simulink model "model_FS_PSH_IEEE39"  (R2020b)
settings: Solver=ode3  StartTime=0.0  StopTime=300  FixedStep=Ts  RelTol=1e-3
PostLoadFcn:
  | IEEE39BusLineLength;
  | vNomHV = 345E3;fNom=60;load('Dynamicload.mat');
InitFcn:
  | IEEE39BusLineLength;
  | vNomHV = 345E3;fNom=60;load('Dynamicload.mat');
values from neighbouring files (symbols this model uses):
  Rp = 0.05    [IEEE39BusLineLength.m]
  t_sw_off = 220    [MAIN_FS_PSH_IEEE39.m]    (also in MAIN_T_PSH_IEEE39.m; MAIN_VS_PSH.m = 45)
  t_sw_on = 130    [MAIN_FS_PSH_IEEE39.m]    (also in MAIN_T_PSH_IEEE39.m; MAIN_VS_PSH.m = 35)
  TL_10_11_len = 14    [IEEE39BusLineLength.m]
  TL_10_13_len = 14    [IEEE39BusLineLength.m]
  TL_13_14_len = 32    [IEEE39BusLineLength.m]
  TL_14_15_len = 70    [IEEE39BusLineLength.m]
  TL_15_16_len = 31.5    [IEEE39BusLineLength.m]
  TL_16_17_len = 26    [IEEE39BusLineLength.m]
  TL_16_19_len = 61    [IEEE39BusLineLength.m]
  TL_16_21_len = 46    [IEEE39BusLineLength.m]
  TL_16_24_len = 15    [IEEE39BusLineLength.m]
  TL_17_18_len = 26    [IEEE39BusLineLength.m]
  TL_17_27_len = 59    [IEEE39BusLineLength.m]
  TL_1_2_len = 134    [IEEE39BusLineLength.m]
  TL_1_39_len = 105    [IEEE39BusLineLength.m]
  TL_21_22_len = 47    [IEEE39BusLineLength.m]
  TL_22_23_len = 33    [IEEE39BusLineLength.m]
  TL_24_23_len = 88    [IEEE39BusLineLength.m]
  TL_25_26_len = 101    [IEEE39BusLineLength.m]
  TL_26_27_len = 46.5    [IEEE39BusLineLength.m]
  TL_26_28_len = 151    [IEEE39BusLineLength.m]
  TL_26_29_len = 200    [IEEE39BusLineLength.m]
  TL_28_29_len = 48    [IEEE39BusLineLength.m]
  TL_2_25_len = 28    [IEEE39BusLineLength.m]
  TL_2_2_len = 49    [IEEE39BusLineLength.m]
  TL_3_18_len = 42    [IEEE39BusLineLength.m]
  TL_3_4_len = 53    [IEEE39BusLineLength.m]
  TL_4_14_len = 33    [IEEE39BusLineLength.m]
  TL_4_5_len = 32.5    [IEEE39BusLineLength.m]
  TL_5_6_len = 14    [IEEE39BusLineLength.m]
  TL_5_8_len = 32    [IEEE39BusLineLength.m]
  TL_6_11_len = 26.5    [IEEE39BusLineLength.m]
  TL_6_7_len = 25.5    [IEEE39BusLineLength.m]
  TL_7_8_len = 15    [IEEE39BusLineLength.m]
  TL_8_9_len = 93    [IEEE39BusLineLength.m]
  TL_9_39_len = 136    [IEEE39BusLineLength.m]
  Ts = 25e-6    (= 2.5e-05)    [MAIN_FS_PSH_IEEE39.m]    (also in MAIN_T_PSH_IEEE39.m; MAIN_VS_PSH.m = 1e-07)
undefined symbols (not defined in the file or in its folder): D1, Delta, FS_PSH, load15, load16, load18, load20, load21, load23, load24, load25, load26, load27, load28, load29, load3, load39, load4, load7, load8
libraries: powerlib x216, sps_avr x10, powerlib_meascontrol x5, pid_lib x1
(part 6 of 8)

== system model_FS_PSH_IEEE39/SS_EastSystem2/GT 6 ==
  5 MW : powerlib/Elements/Three-Phase Parallel RLC Load  LConnTagsString=A|B|C  Configuration=Y (grounded)  NominalVoltage=22e3  Vabc=[1e3 1e3 1e3]  Vabcp=[1e3 1e3 1e3]  NominalFrequency=fNom  UnbalancedPower=off  ActivePower=5e6  InductivePower=0  CapacitivePower=0  Pabc=[10e3 9e3 11e3]  QLabc=[100 90 110]  QCabc=[100 90 110]  Pabcp=[10e3 9e3 11e3]  QLabcp=[100 90 110]  QCabcp=[100 90 110]  Measurements=None  LoadType=constant Z
  Bus Selector1 : BusSelector  OutputSignals="dq0 components.Stator voltage  vq (pu),dq0 components.Stator voltage  vd (pu),Mechanical.Rotor speed  wm  (pu),Mechanical.Rotor speed deviation  dw (pu),Output active power   Peo (pu),Output reactive power  Qeo (pu)"
  Bus 35 : powerlib/Measurements/Three-Phase V-I Measurement  VoltageMeasurement=phase-to-ground  SetLabelV=on  LabelV=V_bus_G6  Vpu=off  VpuLL=off  CurrentMeasurement=no  SetLabelI=on  LabelI=I_bus_G6  Ipu=off  Pbase=100e6  Vbase=16.5e3  OutputType=Complex  PhasorSimulation=off  PSBequivalent=0
  Excitation System : sps_avr/Excitation System  tr=20e-3  reg=[ 200, 0.02 ]  exc=[ 1, 0 .19]  tgr=[ 0, 0 ]  damp=[ 0.0012, 1 ]  sat=[ 0, 0 ]  lim=[ 0, 7.32, 0 ]  v0=[1.02 1.8033]
      settings: SourceProductBaseCode=PS
  GT1_CB8 : Subsystem
  Ground : Ground
  HTG : powerlib/Machines/Hydraulic Turbine and Governor  sm="[ 10/3  0.07 ]"  gate="[  0.01  0.97518  -0.1  0.1 ]"  reg="[  Rp  1.163  0.105  0  0.01  ]"  hyd="[  0  2.67  ]"  dref=0  po=0.51
      settings: SourceProductBaseCode=PS
  Load Flow Bus : powerlib/Measurements/Load Flow Bus  LConnTagsString=a  Phases=single  Connectors=on one side  ID=Bus-35  Vbase=22000  Vref=1.02  Vangle=0  VLF=1.02  VLFb=1  VLFc=1  angleLF=-1.943  angleLFb=0  angleLFc=0
      settings: AttributesFormatString=%<ID>\n%<Vbase>V\n%<VLF>pu\n%<angleLF>deg.
  Machine 6 1000 MVA 22 kV : powerlib/Machines/Synchronous Machine pu Standard  PresetModel=No  MechanicalLoad=Mechanical power Pm  ShowDetailedParameters=on  RotorType=Round  Units=per unit standard parameters  MeasurementBus=off  NominalParameters="[ 1000E6  22000   fNom]"  Reactances1=[ 2.032 0.4 0.2 1.928 0.651 0.2 0.022 ]  Reactances2=[ 0.995, 0.195, 0.155, 0.568, 0.143, 0.16 ]  dAxisTimeConstants=Open-circuit  qAxisTimeConstants=Open-circuit  TimeConstants1=[]  TimeConstants2=[7.3 0.03 0.4 0.04]  TimeConstants3=[]  TimeConstants4=[]  TimeConstants5=[ 9.2, 0.01, 0.01 ]  TimeConstants6=[]  TimeConstants7=[]  TimeConstants8=[]  StatorResistance=0.005  Mechanical=[ 4.35 0.02 20]  PolePairs=20  InitialConditions=[0 -55.6147 0.575854 0.575854 0.575854 -22.492 -142.492 97.508 1.80331]  SetSaturation=off  Saturation=[0.6404,0.7127,0.8441,0.9214,0.9956,1.082,1.19,1.316,1.457;0.7,0.7698,0.8872,0.9466,0.9969,1.046,1.1,1.151,1.201]  LoadFlowParameters=[1 650000000 23084.6 0]  TsPowergui=0  TsBlock=-1  IterativeModel=Trapezoidal non iterative  IterativeDiscreteModel=Trapezoidal non iterative  BusType=PV  Pref=5.50e+008  Qref=0  Qmin=-500e6  Qmax=250e6  PLF=0  QLF=0
      settings: AttributesFormatString=\n\n
  Pref : Constant  Value=0.51
  Terminator5 : Terminator
  Transformer 6 880 MVA 22  kV / 345 kV : powerlib/Elements/Three-Phase Transformer (Two Windings)  Winding1Connection=Delta (D1)  Winding2Connection=Yg  CoreType=Three single-phase transformers  SetSaturation=off  Hysteresis=off  DataFile='hysteresis'  SetInitialFlux=off  Measurements=None  UNITS=pu  NominalPower=[ 880e6 fNom]  Winding1="[ 22e3  0.0   0.0143*880/100/2]"  Winding2="[ 1.025*345e3 0.0   0.0143*880/100/2]"  Rm=500  Lm=500  L0=0.5  Saturation="[ 0,0  ;  0.005,1.2  ;  1.0,1.4 ]"  InitialFluxes=[ 0.8 , -0.8 , 0.7 ]  BreakLoop=off  DiscreteSolver=Trapezoidal iterative  DataType=off  TransfoNumber=0
  Vref : Constant  Value=1.02
  wref : Constant
  A : PMIOPort  Side=Right
  B : PMIOPort  Port=2  Side=Right
  C : PMIOPort  Port=3  Side=Right
  tag scope: P_G6=global, Q_G6=global, V_G6=global, Wm_G6=global
  wires:
  Ground/1 -> Excitation System/4
  HTG/2 -> Terminator5/1
  Vref/1 -> Excitation System/1
  Pref/1 -> HTG/2
  wref/1 -> HTG/1
  Excitation System/1 -> Machine 6 1000 MVA 22 kV/2
  HTG/1 -> Machine 6 1000 MVA 22 kV/1
  Machine 6 1000 MVA 22 kV/1 -> Bus Selector1/1
  Bus Selector1/1 -> Excitation System/3  "<Stator voltage  vq (pu)>"
  Bus Selector1/2 -> Excitation System/2  "<Stator voltage  vd (pu)>"
  Bus Selector1/3 -> HTG/3, [Wm_G6]  "<Rotor speed  wm  (pu)>"
  Bus Selector1/4 -> HTG/5  "<Rotor speed deviation  dw (pu)>"
  Bus Selector1/5 -> HTG/4, [P_G6]  "<Output active power   Peo (pu)>"
  Bus Selector1/6 -> [Q_G6]  "<Output reactive power  Qeo (pu)>"
  [V_bus_G6] -> [V_G6]
  connections:
  Transformer 6 880 MVA 22  kV / 345 kV/LConn1 -- Load Flow Bus/LConn1 -- Bus 35/RConn1 -- 5 MW/LConn1
  Transformer 6 880 MVA 22  kV / 345 kV/LConn2 -- Bus 35/RConn2 -- 5 MW/LConn2
  Transformer 6 880 MVA 22  kV / 345 kV/LConn3 -- Bus 35/RConn3 -- 5 MW/LConn3
  Machine 6 1000 MVA 22 kV/RConn1 -- Bus 35/LConn1
  Machine 6 1000 MVA 22 kV/RConn2 -- Bus 35/LConn2
  Machine 6 1000 MVA 22 kV/RConn3 -- Bus 35/LConn3
  GT1_CB8/LConn1 -- Transformer 6 880 MVA 22  kV / 345 kV/RConn1
  GT1_CB8/LConn2 -- Transformer 6 880 MVA 22  kV / 345 kV/RConn2
  GT1_CB8/LConn3 -- Transformer 6 880 MVA 22  kV / 345 kV/RConn3
  B/RConn1 -- GT1_CB8/RConn2
  A/RConn1 -- GT1_CB8/RConn1
  C/RConn1 -- GT1_CB8/RConn3

== system model_FS_PSH_IEEE39/SS_EastSystem2/GT 7 ==
  5 MW : powerlib/Elements/Three-Phase Parallel RLC Load  LConnTagsString=A|B|C  Configuration=Y (grounded)  NominalVoltage=22e3  Vabc=[1e3 1e3 1e3]  Vabcp=[1e3 1e3 1e3]  NominalFrequency=fNom  UnbalancedPower=off  ActivePower=5e6  InductivePower=0  CapacitivePower=0  Pabc=[10e3 9e3 11e3]  QLabc=[100 90 110]  QCabc=[100 90 110]  Pabcp=[10e3 9e3 11e3]  QLabcp=[100 90 110]  QCabcp=[100 90 110]  Measurements=None  LoadType=constant Z
  Bus Selector1 : BusSelector  OutputSignals="dq0 components.Stator voltage  vq (pu),dq0 components.Stator voltage  vd (pu),Mechanical.Rotor speed  wm  (pu),Mechanical.Rotor speed deviation  dw (pu),Output active power   Peo (pu),Output reactive power  Qeo (pu)"
  Bus 36 : powerlib/Measurements/Three-Phase V-I Measurement  VoltageMeasurement=phase-to-ground  SetLabelV=on  LabelV=V_bus_G7  Vpu=off  VpuLL=off  CurrentMeasurement=no  SetLabelI=on  LabelI=I_bus_G7  Ipu=off  Pbase=100e6  Vbase=16.5e3  OutputType=Complex  PhasorSimulation=off  PSBequivalent=0
  Excitation System : sps_avr/Excitation System  tr=20e-3  reg=[ 200, 0.02 ]  exc=[ 1, 0 .19]  tgr=[ 0, 0 ]  damp=[ 0.0012, 1 ]  sat=[ 0, 0 ]  lim=[ 0, 7.32, 0 ]  v0=[1.015 1.5412]
      settings: SourceProductBaseCode=PS
  GT1_CB10 : Subsystem
  Ground : Ground
  HTG : powerlib/Machines/Hydraulic Turbine and Governor  sm="[ 10/3  0.07 ]"  gate="[  0.01  0.97518  -0.1  0.1 ]"  reg="[  Rp  1.163  0.105  0  0.01  ]"  hyd="[  0  2.67  ]"  dref=0  po=0.42
      settings: SourceProductBaseCode=PS
  Load Flow Bus : powerlib/Measurements/Load Flow Bus  LConnTagsString=a  Phases=single  Connectors=on one side  ID=Bus-36  Vbase=22000  Vref=1.015  Vangle=0  VLF=1.015  VLFb=1  VLFc=1  angleLF=0.3154  angleLFb=0  angleLFc=0
      settings: AttributesFormatString=%<ID>\n%<Vbase>V\n%<VLF>pu\n%<angleLF>deg.
  Machine 7 1000 MVA 22 kV : powerlib/Machines/Synchronous Machine pu Standard  PresetModel=No  MechanicalLoad=Mechanical power Pm  ShowDetailedParameters=on  RotorType=Round  Units=per unit standard parameters  MeasurementBus=off  NominalParameters="[ 1000E6  22000   fNom]"  Reactances1=[ 2.408 0.4 0.2 2.384 1.518 0.2 0.032 ]  Reactances2=[ 0.995, 0.195, 0.155, 0.568, 0.143, 0.16 ]  dAxisTimeConstants=Open-circuit  qAxisTimeConstants=Open-circuit  TimeConstants1=[]  TimeConstants2=[5.66 0.03 1.5 0.04]  TimeConstants3=[]  TimeConstants4=[]  TimeConstants5=[ 9.2, 0.01, 0.01 ]  TimeConstants6=[]  TimeConstants7=[]  TimeConstants8=[]  StatorResistance=0.005  Mechanical=[ 3.23 0.02 20]  PolePairs=20  InitialConditions=[0 -44.8827 0.454166 0.454166 0.454166 -3.41889 -123.419 116.581 1.54123]  SetSaturation=off  Saturation=[0.6404,0.7127,0.8441,0.9214,0.9956,1.082,1.19,1.316,1.457;0.7,0.7698,0.8872,0.9466,0.9969,1.046,1.1,1.151,1.201]  LoadFlowParameters=[1 560000000 23397 0]  TsPowergui=0  TsBlock=-1  IterativeModel=Trapezoidal non iterative  IterativeDiscreteModel=Trapezoidal non iterative  BusType=PV  Pref=4.6e+008  Qref=0  Qmin=-500e6  Qmax=150e6  PLF=0  QLF=0
      settings: AttributesFormatString=\n\n
  Pref : Constant  Value=0.42
  Terminator5 : Terminator
  Transformer 6 880 MVA 22  kV / 345 kV : powerlib/Elements/Three-Phase Transformer (Two Windings)  Winding1Connection=Delta (D1)  Winding2Connection=Yg  CoreType=Three single-phase transformers  SetSaturation=off  Hysteresis=off  DataFile='hysteresis'  SetInitialFlux=off  Measurements=None  UNITS=pu  NominalPower=[ 897.6e6 fNom]  Winding1="[ 22e3  0.0   0.0143*880/100/2]"  Winding2="[ 1.025*345e3 0.0   0.0143*880/100/2]"  Rm=500  Lm=500  L0=0.5  Saturation="[ 0,0  ;  0.005,1.2  ;  1.0,1.4 ]"  InitialFluxes=[ 0.8 , -0.8 , 0.7 ]  BreakLoop=off  DiscreteSolver=Trapezoidal iterative  DataType=off  TransfoNumber=0
  Vref : Constant  Value=1.015
  wref : Constant
  A : PMIOPort  Side=Right
  B : PMIOPort  Port=2  Side=Right
  C : PMIOPort  Port=3  Side=Right
  tag scope: P_G7=global, Q_G7=global, V_G7=global, Wm_G7=global
  wires:
  Ground/1 -> Excitation System/4
  HTG/2 -> Terminator5/1
  Vref/1 -> Excitation System/1
  Pref/1 -> HTG/2
  wref/1 -> HTG/1
  Excitation System/1 -> Machine 7 1000 MVA 22 kV/2
  HTG/1 -> Machine 7 1000 MVA 22 kV/1
  Machine 7 1000 MVA 22 kV/1 -> Bus Selector1/1
  Bus Selector1/1 -> Excitation System/3  "<Stator voltage  vq (pu)>"
  Bus Selector1/2 -> Excitation System/2  "<Stator voltage  vd (pu)>"
  Bus Selector1/3 -> HTG/3, [Wm_G7]  "<Rotor speed  wm  (pu)>"
  Bus Selector1/4 -> HTG/5  "<Rotor speed deviation  dw (pu)>"
  Bus Selector1/5 -> HTG/4, [P_G7]  "<Output active power   Peo (pu)>"
  Bus Selector1/6 -> [Q_G7]  "<Output reactive power  Qeo (pu)>"
  [V_bus_G7] -> [V_G7]
  connections:
  Load Flow Bus/LConn1 -- Transformer 6 880 MVA 22  kV / 345 kV/LConn1 -- Bus 36/RConn1 -- 5 MW/LConn1
  Bus 36/RConn2 -- Transformer 6 880 MVA 22  kV / 345 kV/LConn2 -- 5 MW/LConn2
  Bus 36/RConn3 -- Transformer 6 880 MVA 22  kV / 345 kV/LConn3 -- 5 MW/LConn3
  Machine 7 1000 MVA 22 kV/RConn1 -- Bus 36/LConn1
  Machine 7 1000 MVA 22 kV/RConn2 -- Bus 36/LConn2
  Machine 7 1000 MVA 22 kV/RConn3 -- Bus 36/LConn3
  Transformer 6 880 MVA 22  kV / 345 kV/RConn3 -- GT1_CB10/LConn3
  Transformer 6 880 MVA 22  kV / 345 kV/RConn2 -- GT1_CB10/LConn2
  Transformer 6 880 MVA 22  kV / 345 kV/RConn1 -- GT1_CB10/LConn1
  B/RConn1 -- GT1_CB10/RConn2
  A/RConn1 -- GT1_CB10/RConn1
  C/RConn1 -- GT1_CB10/RConn3

== system model_FS_PSH_IEEE39/SS_EastSystem2/Load 21 ==
  Bus_L21 : powerlib/Measurements/Three-Phase V-I Measurement  VoltageMeasurement=phase-to-ground  SetLabelV=off  LabelV=V_Bus_L21  Vpu=off  VpuLL=off  CurrentMeasurement=yes  SetLabelI=on  LabelI=I_L21  Ipu=off  Pbase=100e6  Vbase=230e3  OutputType=Complex  PhasorSimulation=off  PSBequivalent=0
  Terminator : Terminator
  Three-Phase Dynamic Load : powerlib/Elements/Three-Phase Dynamic Load  NominalVoltage=[345e3 fNom]  ActiveReactivePowers=[2.74e+08 1.15e+08]  PositiveSequence=[1.00586 20.5637]  ExternalControl=on  NpNq=[0 0]  TimeConstants="[0  0  0  0]"  MinimumVoltage=0.7  Tfilter=1e-4  LoadFlowParameters=[4,0,0,0,0]
      settings: SourceProductBaseCode=PS
  A : PMIOPort  Side=Left
  B : PMIOPort  Port=2  Side=Left
  C : PMIOPort  Port=3  Side=Left
  tag scope: V_L21=global
  wires:
  Three-Phase Dynamic Load/1 -> Terminator/1
  Bus_L21/1 -> [V_L21]
  [load21] -> Three-Phase Dynamic Load/1
  connections:
  Bus_L21/RConn1 -- Three-Phase Dynamic Load/LConn1
  C/RConn1 -- Bus_L21/LConn3
  B/RConn1 -- Bus_L21/LConn2
  A/RConn1 -- Bus_L21/LConn1
  Bus_L21/RConn2 -- Three-Phase Dynamic Load/LConn2
  Bus_L21/RConn3 -- Three-Phase Dynamic Load/LConn3

== system model_FS_PSH_IEEE39/SS_EastSystem2/Load 23 ==
  Bus_L23 : powerlib/Measurements/Three-Phase V-I Measurement  VoltageMeasurement=phase-to-ground  SetLabelV=off  LabelV=V_Bus_L23  Vpu=off  VpuLL=off  CurrentMeasurement=yes  SetLabelI=on  LabelI=I_L23  Ipu=off  Pbase=100e6  Vbase=230e3  OutputType=Complex  PhasorSimulation=off  PSBequivalent=0
  Terminator : Terminator
  Three-Phase Dynamic Load : powerlib/Elements/Three-Phase Dynamic Load  NominalVoltage=[345e3 fNom]  ActiveReactivePowers=[2.475e+08 8.46e+07]  PositiveSequence=[1.0123 23.421]  ExternalControl=on  NpNq=[0 0]  TimeConstants="[0  0  0  0]"  MinimumVoltage=0.7  Tfilter=1e-4  LoadFlowParameters=[4,0,0,0,0]
      settings: SourceProductBaseCode=PS
  A : PMIOPort  Side=Left
  B : PMIOPort  Port=2  Side=Left
  C : PMIOPort  Port=3  Side=Left
  tag scope: V_L23=global
  wires:
  Three-Phase Dynamic Load/1 -> Terminator/1
  Bus_L23/1 -> [V_L23]
  [load23] -> Three-Phase Dynamic Load/1
  connections:
  Three-Phase Dynamic Load/LConn1 -- Bus_L23/RConn1
  C/RConn1 -- Bus_L23/LConn3
  B/RConn1 -- Bus_L23/LConn2
  A/RConn1 -- Bus_L23/LConn1
  Three-Phase Dynamic Load/LConn2 -- Bus_L23/RConn2
  Three-Phase Dynamic Load/LConn3 -- Bus_L23/RConn3

== system model_FS_PSH_IEEE39/SS_EastSystem2/Load 24 ==
  Bus_L24 : powerlib/Measurements/Three-Phase V-I Measurement  VoltageMeasurement=phase-to-ground  SetLabelV=off  LabelV=V_Bus_L24  Vpu=off  VpuLL=off  CurrentMeasurement=yes  SetLabelI=on  LabelI=I_L24  Ipu=off  Pbase=100e6  Vbase=230e3  OutputType=Complex  PhasorSimulation=off  PSBequivalent=0
  Terminator : Terminator
  Three-Phase Dynamic Load : powerlib/Elements/Three-Phase Dynamic Load  NominalVoltage=[345e3 fNom]  ActiveReactivePowers=[3.086e+08 -9.2e+07]  PositiveSequence=[1.01137 19.0799]  ExternalControl=on  NpNq=[0 0]  TimeConstants="[0  0  0  0]"  MinimumVoltage=0.7  Tfilter=1e-4  LoadFlowParameters=[4,0,0,0,0]
      settings: SourceProductBaseCode=PS
  A : PMIOPort  Side=Left
  B : PMIOPort  Port=2  Side=Left
  C : PMIOPort  Port=3  Side=Left
  tag scope: V_L24=global
  wires:
  Three-Phase Dynamic Load/1 -> Terminator/1
  Bus_L24/1 -> [V_L24]
  [load24] -> Three-Phase Dynamic Load/1
  connections:
  Three-Phase Dynamic Load/LConn3 -- Bus_L24/RConn3
  Three-Phase Dynamic Load/LConn2 -- Bus_L24/RConn2
  A/RConn1 -- Bus_L24/LConn1
  B/RConn1 -- Bus_L24/LConn2
  C/RConn1 -- Bus_L24/LConn3
  Three-Phase Dynamic Load/LConn1 -- Bus_L24/RConn1

== system model_FS_PSH_IEEE39/SS_EastSystem2/Machines Measurements ==
  Mux : Mux  Inputs=2
  Mux3 : Mux
  Mux4 : Mux
  Machines Measurements : Outport
  wires:
  Mux4/1 -> Mux/2
  Mux3/1 -> Mux/1
  [Wm_G7] -> Mux4/4
  [Q_G7] -> Mux4/3
  [P_G7] -> Mux4/2
  [V_G7] -> Mux4/1
  [Wm_G6] -> Mux3/4
  [Q_G6] -> Mux3/3
  [P_G6] -> Mux3/2
  [V_G6] -> Mux3/1
  Mux/1 -> Machines Measurements/1

== system model_FS_PSH_IEEE39/SS_NorthSystem1/Buses current_N ==
  Mux3 : Mux
  curremt : Outport
  wires:
  [I_L25] -> Mux3/1
  [I_L26] -> Mux3/2
  [I_L28] -> Mux3/3
  [I_L29] -> Mux3/4
  Mux3/1 -> curremt/1

== system model_FS_PSH_IEEE39/SS_NorthSystem1/Buses voltages_N ==
  Mux3 : Mux
  Voltages : Outport
  wires:
  Mux3/1 -> Voltages/1
  [V_L25] -> Mux3/1
  [V_L26] -> Mux3/2
  [V_L28] -> Mux3/3
  [V_L29] -> Mux3/4

== system model_FS_PSH_IEEE39/SS_NorthSystem1/GT 8 ==
  5 MW : powerlib/Elements/Three-Phase Parallel RLC Load  LConnTagsString=A|B|C  Configuration=Y (grounded)  NominalVoltage=22e3  Vabc=[1e3 1e3 1e3]  Vabcp=[1e3 1e3 1e3]  NominalFrequency=fNom  UnbalancedPower=off  ActivePower=5e6  InductivePower=0  CapacitivePower=0  Pabc=[10e3 9e3 11e3]  QLabc=[100 90 110]  QCabc=[100 90 110]  Pabcp=[10e3 9e3 11e3]  QLabcp=[100 90 110]  QCabcp=[100 90 110]  Measurements=None  LoadType=constant Z
  Bus Selector1 : BusSelector  OutputSignals="dq0 components.Stator voltage  vq (pu),dq0 components.Stator voltage  vd (pu),Mechanical.Rotor speed  wm  (pu),Mechanical.Rotor speed deviation  dw (pu),Output active power   Peo (pu),Output reactive power  Qeo (pu)"
  Bus 37 : powerlib/Measurements/Three-Phase V-I Measurement  VoltageMeasurement=phase-to-ground  SetLabelV=on  LabelV=V_bus_G8  Vpu=off  VpuLL=off  CurrentMeasurement=no  SetLabelI=on  LabelI=I_bus_G8  Ipu=off  Pbase=100e6  Vbase=16.5e3  OutputType=Complex  PhasorSimulation=off  PSBequivalent=0
  Excitation System : sps_avr/Excitation System  tr=20e-3  reg=[ 200, 0.02 ]  exc=[ 1, 0 .19]  tgr=[ 0, 0 ]  damp=[ 0.0012, 1 ]  sat=[ 0, 0 ]  lim=[ 0, 7.32, 0 ]  v0=[1.01 1.6849]
      settings: SourceProductBaseCode=PS
  GT1_CB11 : Subsystem
  Ground : Ground
  HTG : powerlib/Machines/Hydraulic Turbine and Governor  sm="[ 10/3  0.07 ]"  gate="[  0.01  0.97518  -0.1  0.1 ]"  reg="[  Rp  1.163  0.105  0  0.01  ]"  hyd="[  0  2.67  ]"  dref=0  po=0.6
      settings: SourceProductBaseCode=PS
  Load Flow Bus : powerlib/Measurements/Load Flow Bus  LConnTagsString=a  Phases=single  Connectors=on one side  ID=Bus-37  Vbase=22000  Vref=1.01  Vangle=0  VLF=1.01  VLFb=1  VLFc=1  angleLF=3.342  angleLFb=0  angleLFc=0
      settings: AttributesFormatString=%<ID>\n%<Vbase>V\n%<VLF>pu\n%<angleLF>deg.
  Machine 8 1000 MVA 22 kV : powerlib/Machines/Synchronous Machine pu Standard  PresetModel=No  MechanicalLoad=Mechanical power Pm  ShowDetailedParameters=on  RotorType=Round  Units=per unit standard parameters  MeasurementBus=off  NominalParameters="[ 1000E6  22000   fNom]"  Reactances1=[ 2.035 0.4 0.2 1.965 0.639 0.2 0.028 ]  Reactances2=[ 0.995, 0.195, 0.155, 0.568, 0.143, 0.16 ]  dAxisTimeConstants=Open-circuit  qAxisTimeConstants=Open-circuit  TimeConstants1=[]  TimeConstants2=[6.7 0.03 0.41 0.04]  TimeConstants3=[]  TimeConstants4=[]  TimeConstants5=[ 9.2, 0.01, 0.01 ]  TimeConstants6=[]  TimeConstants7=[]  TimeConstants8=[]  StatorResistance=0.005  Mechanical=[ 3.46 0.02 20]  PolePairs=20  InitialConditions=[0 -37.6671 0.634647 0.634647 0.634647 0.151083 -119.849 120.151 1.68493]  SetSaturation=off  Saturation=[0.6404,0.7127,0.8441,0.9214,0.9956,1.082,1.19,1.316,1.457;0.7,0.7698,0.8872,0.9466,0.9969,1.046,1.1,1.151,1.201]  LoadFlowParameters=[1 540000000 22611.6 0]  TsPowergui=0  TsBlock=-1  IterativeModel=Trapezoidal non iterative  IterativeDiscreteModel=Trapezoidal non iterative  BusType=PV  Pref=6.4e+008  Qref=0  Qmin=-500e6  Qmax=50e6  PLF=0  QLF=0
      settings: AttributesFormatString=\n\n
  Pref : Constant  Value=0.6
  Terminator5 : Terminator
  Transformer 8 772.2 MVA 22 kV / 345 kV : powerlib/Elements/Three-Phase Transformer (Two Windings)  Winding1Connection=Delta (D1)  Winding2Connection=Yg  CoreType=Three single-phase transformers  SetSaturation=off  Hysteresis=off  DataFile='hysteresis'  SetInitialFlux=off  Measurements=None  UNITS=pu  NominalPower=[ 1000e6 fNom]  Winding1="[ 22e3    0.0006*1000/100/2  0.0232*1000/100/2 ]"  Winding2="[ 1.025*345e3    0.0006*1000/100/2  0.0232*1000/100/2  ]"  Rm=500  Lm=500  L0=0.5  Saturation="[ 0,0  ;  0.005,1.2  ;  1.0,1.4 ]"  InitialFluxes=[ 0.8 , -0.8 , 0.7 ]  BreakLoop=off  DiscreteSolver=Trapezoidal iterative  DataType=off  TransfoNumber=0
  Vref : Constant  Value=1.01
  wref : Constant
  A : PMIOPort  Side=Right
  B : PMIOPort  Port=2  Side=Right
  C : PMIOPort  Port=3  Side=Right
  tag scope: P_G8=global, Q_G8=global, V_G8=global, Wm_G8=global
  wires:
  [V_bus_G8] -> [V_G8]
  Bus Selector1/6 -> [Q_G8]  "<Output reactive power  Qeo (pu)>"
  Bus Selector1/5 -> [P_G8], HTG/4  "<Output active power   Peo (pu)>"
  Bus Selector1/4 -> HTG/5  "<Rotor speed deviation  dw (pu)>"
  Bus Selector1/3 -> [Wm_G8], HTG/3  "<Rotor speed  wm  (pu)>"
  Bus Selector1/2 -> Excitation System/2  "<Stator voltage  vd (pu)>"
  Bus Selector1/1 -> Excitation System/3  "<Stator voltage  vq (pu)>"
  Machine 8 1000 MVA 22 kV/1 -> Bus Selector1/1
  HTG/1 -> Machine 8 1000 MVA 22 kV/1
  Excitation System/1 -> Machine 8 1000 MVA 22 kV/2
  wref/1 -> HTG/1
  Pref/1 -> HTG/2
  Vref/1 -> Excitation System/1
  HTG/2 -> Terminator5/1
  Ground/1 -> Excitation System/4
  connections:
  Machine 8 1000 MVA 22 kV/RConn3 -- Bus 37/LConn3
  Machine 8 1000 MVA 22 kV/RConn2 -- Bus 37/LConn2
  Machine 8 1000 MVA 22 kV/RConn1 -- Bus 37/LConn1
  5 MW/LConn3 -- Bus 37/RConn3 -- Transformer 8 772.2 MVA 22 kV / 345 kV/LConn3
  5 MW/LConn2 -- Bus 37/RConn2 -- Transformer 8 772.2 MVA 22 kV / 345 kV/LConn2
  5 MW/LConn1 -- Bus 37/RConn1 -- Load Flow Bus/LConn1 -- Transformer 8 772.2 MVA 22 kV / 345 kV/LConn1
  GT1_CB11/LConn1 -- Transformer 8 772.2 MVA 22 kV / 345 kV/RConn1
  GT1_CB11/LConn2 -- Transformer 8 772.2 MVA 22 kV / 345 kV/RConn2
  GT1_CB11/LConn3 -- Transformer 8 772.2 MVA 22 kV / 345 kV/RConn3
  C/RConn1 -- GT1_CB11/RConn3
  B/RConn1 -- GT1_CB11/RConn2
  A/RConn1 -- GT1_CB11/RConn1

== system model_FS_PSH_IEEE39/SS_NorthSystem1/GT 9 ==
  5 MW : powerlib/Elements/Three-Phase Parallel RLC Load  LConnTagsString=A|B|C  Configuration=Y (grounded)  NominalVoltage=22e3  Vabc=[1e3 1e3 1e3]  Vabcp=[1e3 1e3 1e3]  NominalFrequency=fNom  UnbalancedPower=off  ActivePower=5e6  InductivePower=0  CapacitivePower=0  Pabc=[10e3 9e3 11e3]  QLabc=[100 90 110]  QCabc=[100 90 110]  Pabcp=[10e3 9e3 11e3]  QLabcp=[100 90 110]  QCabcp=[100 90 110]  Measurements=None  LoadType=constant Z
  Bus Selector1 : BusSelector  OutputSignals="dq0 components.Stator voltage  vq (pu),dq0 components.Stator voltage  vd (pu),Mechanical.Rotor speed  wm  (pu),Mechanical.Rotor speed deviation  dw (pu),Output active power   Peo (pu),Output reactive power  Qeo (pu)"
  Bus 38 : powerlib/Measurements/Three-Phase V-I Measurement  VoltageMeasurement=phase-to-ground  SetLabelV=on  LabelV=V_bus_G9  Vpu=off  VpuLL=off  CurrentMeasurement=no  SetLabelI=on  LabelI=I_bus_G9  Ipu=off  Pbase=100e6  Vbase=16.5e3  OutputType=Complex  PhasorSimulation=off  PSBequivalent=0
  Excitation System : sps_avr/Excitation System  tr=20e-3  reg=[ 200, 0.02 ]  exc=[ 1, 0 .19]  tgr=[ 0, 0 ]  damp=[ 0.0012, 1 ]  sat=[ 0, 0 ]  lim=[ 0, 7.32, 0 ]  v0=[1.0156 1.6973]
      settings: SourceProductBaseCode=PS
  GT1_CB12 : Subsystem
  Ground : Ground
  HTG : powerlib/Machines/Hydraulic Turbine and Governor  sm="[ 10/3  0.07 ]"  gate="[  0.01  0.97518  -0.1  0.1 ]"  reg="[  Rp  1.163  0.105  0  0.01  ]"  hyd="[  0  2.67  ]"  dref=0  po=0.654
      settings: SourceProductBaseCode=PS
  Load Flow Bus : powerlib/Measurements/Load Flow Bus  LConnTagsString=a  Phases=single  Connectors=on one side  ID=Bus-38  Vbase=22000  Vref=1.0265  Vangle=0  VLF=1.016  VLFb=1  VLFc=1  angleLF=1.986  angleLFb=0  angleLFc=0
      settings: AttributesFormatString=%<ID>\n%<Vbase>V\n%<VLF>pu\n%<angleLF>deg.
  Machine 9 1000 MVA 22 kV : powerlib/Machines/Synchronous Machine pu Standard  PresetModel=No  MechanicalLoad=Mechanical power Pm  ShowDetailedParameters=on  RotorType=Round  Units=per unit standard parameters  MeasurementBus=off  NominalParameters="[ 1000E6  22000   fNom]"  Reactances1=[ 1.7901 0.4845 0.242 1.742 0.4989 0.242 0.03 ]  Reactances2=[ 0.995, 0.195, 0.155, 0.568, 0.143, 0.16 ]  dAxisTimeConstants=Open-circuit  qAxisTimeConstants=Open-circuit  TimeConstants1=[]  TimeConstants2=[4.79 0.03 1.96 0.04]  TimeConstants3=[]  TimeConstants4=[]  TimeConstants5=[ 9.2, 0.01, 0.01 ]  TimeConstants6=[]  TimeConstants7=[]  TimeConstants8=[]  StatorResistance=0.005  Mechanical=[ 4.058 0.02 20]  PolePairs=20  InitialConditions=[0 -39.4462 0.720476 0.720476 0.720476 -1.93203 -121.932 118.068 1.69726]  SetSaturation=off  Saturation=[0.6404,0.7127,0.8441,0.9214,0.9956,1.082,1.19,1.316,1.457;0.7,0.7698,0.8872,0.9466,0.9969,1.046,1.1,1.151,1.201]  LoadFlowParameters=[1 830000000 22583 0]  TsPowergui=0  TsBlock=-1  IterativeModel=Trapezoidal non iterative  IterativeDiscreteModel=Trapezoidal non iterative  BusType=PV  Pref=7.3e+008  Qref=0  Qmin=-500e6  Qmax=50e6  PLF=0  QLF=0
      settings: AttributesFormatString=\n\n
  Terminator5 : Terminator
  Transformer 9 935 MVA 22 kV / 345 kV : powerlib/Elements/Three-Phase Transformer (Two Windings)  Winding1Connection=Delta (D1)  Winding2Connection=Yg  CoreType=Three single-phase transformers  SetSaturation=off  Hysteresis=off  DataFile='hysteresis'  SetInitialFlux=off  Measurements=None  UNITS=pu  NominalPower=[ 935e6 fNom]  Winding1="[ 22e3  0.0008*935/100/2  0.0156*935/100/2]"  Winding2="[ 1.025*345e3  0.0008*935/100/2  0.0156*935/100/2]"  Rm=500  Lm=500  L0=0.5  Saturation="[ 0,0  ;  0.005,1.2  ;  1.0,1.4 ]"  InitialFluxes=[ 0.8 , -0.8 , 0.7 ]  BreakLoop=off  DiscreteSolver=Trapezoidal iterative  DataType=off  TransfoNumber=0
  wref : Constant
  wref1 : Constant  Value=0.654
  wref2 : Constant  Value=1.0265
  A : PMIOPort  Side=Right
  B : PMIOPort  Port=2  Side=Right
  C : PMIOPort  Port=3  Side=Right
  tag scope: P_G9=global, Q_G9=global, V_G9=global, Wm_G9=global
  wires:
  Ground/1 -> Excitation System/4
  HTG/2 -> Terminator5/1
  wref2/1 -> Excitation System/1
  wref1/1 -> HTG/2
  wref/1 -> HTG/1
  Excitation System/1 -> Machine 9 1000 MVA 22 kV/2
  HTG/1 -> Machine 9 1000 MVA 22 kV/1
  Machine 9 1000 MVA 22 kV/1 -> Bus Selector1/1
  Bus Selector1/1 -> Excitation System/3  "<Stator voltage  vq (pu)>"
  Bus Selector1/2 -> Excitation System/2  "<Stator voltage  vd (pu)>"
  Bus Selector1/3 -> HTG/3, [Wm_G9]  "<Rotor speed  wm  (pu)>"
  Bus Selector1/4 -> HTG/5  "<Rotor speed deviation  dw (pu)>"
  Bus Selector1/5 -> HTG/4, [P_G9]  "<Output active power   Peo (pu)>"
  Bus Selector1/6 -> [Q_G9]  "<Output reactive power  Qeo (pu)>"
  [V_bus_G9] -> [V_G9]
  connections:
  Transformer 9 935 MVA 22 kV / 345 kV/LConn1 -- Load Flow Bus/LConn1 -- Bus 38/RConn1 -- 5 MW/LConn1
  Transformer 9 935 MVA 22 kV / 345 kV/LConn2 -- Bus 38/RConn2 -- 5 MW/LConn2
  Transformer 9 935 MVA 22 kV / 345 kV/LConn3 -- Bus 38/RConn3 -- 5 MW/LConn3
  Machine 9 1000 MVA 22 kV/RConn1 -- Bus 38/LConn1
  Machine 9 1000 MVA 22 kV/RConn2 -- Bus 38/LConn2
  Machine 9 1000 MVA 22 kV/RConn3 -- Bus 38/LConn3
  Transformer 9 935 MVA 22 kV / 345 kV/RConn2 -- GT1_CB12/LConn2
  Transformer 9 935 MVA 22 kV / 345 kV/RConn1 -- GT1_CB12/LConn1
  Transformer 9 935 MVA 22 kV / 345 kV/RConn3 -- GT1_CB12/LConn3
  B/RConn1 -- GT1_CB12/RConn2
  C/RConn1 -- GT1_CB12/RConn3
  A/RConn1 -- GT1_CB12/RConn1

== system model_FS_PSH_IEEE39/SS_NorthSystem1/Load 25 ==
  Terminator : Terminator
  Three-Phase Dynamic Load : powerlib/Elements/Three-Phase Dynamic Load  NominalVoltage="[345e3  fNom]"  ActiveReactivePowers=[2.24e+08 4.72e+07]  PositiveSequence=[1.03404 25.0543]  ExternalControl=on  NpNq=[0 0]  TimeConstants="[0  0  0  0]"  MinimumVoltage=0.7  Tfilter=1e-4  LoadFlowParameters=[4,0,0,0,0]
      settings: SourceProductBaseCode=PS
  V_Bus_L25 : powerlib/Measurements/Three-Phase V-I Measurement  VoltageMeasurement=phase-to-ground  SetLabelV=off  LabelV=V_Bus_L25  Vpu=off  VpuLL=off  CurrentMeasurement=yes  SetLabelI=on  LabelI=I_L25  Ipu=off  Pbase=100e6  Vbase=230e3  OutputType=Complex  PhasorSimulation=off  PSBequivalent=0
  A : PMIOPort  Side=Left
  B : PMIOPort  Port=2  Side=Left
  C : PMIOPort  Port=3  Side=Left
  tag scope: V_L25=global
  wires:
  Three-Phase Dynamic Load/1 -> Terminator/1
  V_Bus_L25/1 -> [V_L25]
  [load25] -> Three-Phase Dynamic Load/1
  connections:
  V_Bus_L25/RConn1 -- Three-Phase Dynamic Load/LConn1
  C/RConn1 -- V_Bus_L25/LConn3
  B/RConn1 -- V_Bus_L25/LConn2
  A/RConn1 -- V_Bus_L25/LConn1
  V_Bus_L25/RConn2 -- Three-Phase Dynamic Load/LConn2
  V_Bus_L25/RConn3 -- Three-Phase Dynamic Load/LConn3

== system model_FS_PSH_IEEE39/SS_NorthSystem1/Load 26 ==
  Bus_L26 : powerlib/Measurements/Three-Phase V-I Measurement  VoltageMeasurement=phase-to-ground  SetLabelV=off  LabelV=V_Bus_L26  Vpu=off  VpuLL=off  CurrentMeasurement=yes  SetLabelI=on  LabelI=I_L26  Ipu=off  Pbase=100e6  Vbase=230e3  OutputType=Complex  PhasorSimulation=off  PSBequivalent=0
  Terminator : Terminator
  Three-Phase Dynamic Load : powerlib/Elements/Three-Phase Dynamic Load  NominalVoltage=[345e3 fNom]  ActiveReactivePowers=[1.39e+08 1.7e+07]  PositiveSequence=[1.02673 21.7857]  ExternalControl=on  NpNq=[0 0]  TimeConstants="[0  0  0  0]"  MinimumVoltage=0.7  Tfilter=1e-4  LoadFlowParameters=[4,0,0,0,0]
      settings: SourceProductBaseCode=PS
  A : PMIOPort  Side=Left
  B : PMIOPort  Port=2  Side=Left
  C : PMIOPort  Port=3  Side=Left
  tag scope: V_L26=global
  wires:
  Three-Phase Dynamic Load/1 -> Terminator/1
  Bus_L26/1 -> [V_L26]
  [load26] -> Three-Phase Dynamic Load/1
  connections:
  Three-Phase Dynamic Load/LConn1 -- Bus_L26/RConn1
  C/RConn1 -- Bus_L26/LConn3
  B/RConn1 -- Bus_L26/LConn2
  A/RConn1 -- Bus_L26/LConn1
  Bus_L26/RConn2 -- Three-Phase Dynamic Load/LConn2
  Bus_L26/RConn3 -- Three-Phase Dynamic Load/LConn3

== system model_FS_PSH_IEEE39/SS_NorthSystem1/Load 28 ==
  Bus_L28 : powerlib/Measurements/Three-Phase V-I Measurement  VoltageMeasurement=phase-to-ground  SetLabelV=off  LabelV=V_Bus_L28  Vpu=off  VpuLL=off  CurrentMeasurement=yes  SetLabelI=on  LabelI=I_L28  Ipu=off  Pbase=100e6  Vbase=230e3  OutputType=Complex  PhasorSimulation=off  PSBequivalent=0
  Terminator : Terminator
  Three-Phase Dynamic Load : powerlib/Elements/Three-Phase Dynamic Load  NominalVoltage=[345e3 fNom]  ActiveReactivePowers=[2.06e+08 2.76e+07]  PositiveSequence=[1.03092 23.6623]  ExternalControl=on  NpNq=[0 0]  TimeConstants="[0  0  0  0]"  MinimumVoltage=0.7  Tfilter=1e-4  LoadFlowParameters=[4,0,0,0,0]
      settings: SourceProductBaseCode=PS
  A : PMIOPort  Side=Left
  B : PMIOPort  Port=2  Side=Left
  C : PMIOPort  Port=3  Side=Left
  tag scope: V_L28=global
  wires:
  Three-Phase Dynamic Load/1 -> Terminator/1
  Bus_L28/1 -> [V_L28]
  [load28] -> Three-Phase Dynamic Load/1
  connections:
  Bus_L28/RConn3 -- Three-Phase Dynamic Load/LConn3
  Bus_L28/RConn2 -- Three-Phase Dynamic Load/LConn2
  A/RConn1 -- Bus_L28/LConn1
  B/RConn1 -- Bus_L28/LConn2
  C/RConn1 -- Bus_L28/LConn3
  Bus_L28/RConn1 -- Three-Phase Dynamic Load/LConn1

== system model_FS_PSH_IEEE39/SS_NorthSystem1/Load 29 ==
  Bus_L29 : powerlib/Measurements/Three-Phase V-I Measurement  VoltageMeasurement=phase-to-ground  SetLabelV=off  LabelV=V_Bus_L29  Vpu=off  VpuLL=off  CurrentMeasurement=yes  SetLabelI=on  LabelI=I_L29  Ipu=off  Pbase=100e6  Vbase=230e3  OutputType=Complex  PhasorSimulation=off  PSBequivalent=0
  Terminator : Terminator
  Three-Phase Dynamic Load : powerlib/Elements/Three-Phase Dynamic Load  NominalVoltage=[345e3 fNom]  ActiveReactivePowers=[2.835e+08 2.69e+07]  PositiveSequence=[1.03368 25.6776]  ExternalControl=on  NpNq=[0 0]  TimeConstants="[0  0  0  0]"  MinimumVoltage=0.7  Tfilter=1e-4  LoadFlowParameters=[4,0,0,0,0]
      settings: SourceProductBaseCode=PS
  A : PMIOPort  Side=Left
  B : PMIOPort  Port=2  Side=Left
  C : PMIOPort  Port=3  Side=Left
  tag scope: V_L29=global
  wires:
  Three-Phase Dynamic Load/1 -> Terminator/1
  Bus_L29/1 -> [V_L29]
  [load29] -> Three-Phase Dynamic Load/1
  connections:
  Three-Phase Dynamic Load/LConn1 -- Bus_L29/RConn1
  C/RConn1 -- Bus_L29/LConn3
  B/RConn1 -- Bus_L29/LConn2
  A/RConn1 -- Bus_L29/LConn1
  Bus_L29/RConn2 -- Three-Phase Dynamic Load/LConn2
  Bus_L29/RConn3 -- Three-Phase Dynamic Load/LConn3

== system model_FS_PSH_IEEE39/SS_NorthSystem1/Machines Measurements ==
  Mux : Mux  Inputs=2
  Mux1 : Mux
  Mux2 : Mux
  Machines Measurements : Outport
  wires:
  Mux2/1 -> Mux/2
  Mux1/1 -> Mux/1
  Mux/1 -> Machines Measurements/1
  [Wm_G9] -> Mux2/4
  [Q_G9] -> Mux2/3
  [P_G9] -> Mux2/2
  [V_G9] -> Mux2/1
  [Wm_G8] -> Mux1/4
  [Q_G8] -> Mux1/3
  [P_G8] -> Mux1/2
  [V_G8] -> Mux1/1

== system model_FS_PSH_IEEE39/SS_NorthSystem2/Buses current_N ==
  Mux3 : Mux  Inputs=6
  curremt : Outport
  wires:
  [I_bus_1] -> Mux3/1
  [I_bus_2] -> Mux3/2
  [I_L3] -> Mux3/3
  [I_bus_17] -> Mux3/4
  [I_L18] -> Mux3/5
  Mux3/1 -> curremt/1
  [I_L27] -> Mux3/6

== system model_FS_PSH_IEEE39/SS_NorthSystem2/Buses voltages_N ==
  Mux3 : Mux  Inputs=6
  Voltages : Outport
  wires:
  Mux3/1 -> Voltages/1
  [V_L27] -> Mux3/6
  [V_L18] -> Mux3/5
  [V_bus_17] -> Mux3/4
  [V_L3] -> Mux3/3
  [V_bus_2] -> Mux3/2
  [V_bus_1] -> Mux3/1

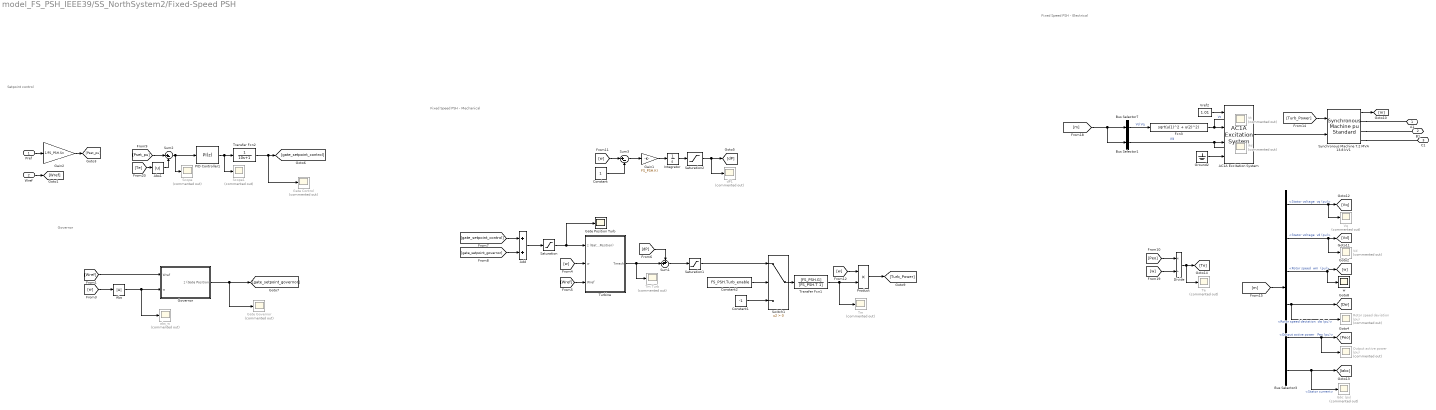
== system model_FS_PSH_IEEE39/SS_NorthSystem2/Fixed-Speed PSH ==
  note: Fixed Speed PSH - Electrical
  note: Fixed Speed PSH - Mechanical
  note: Setpoint control
  note: Governor
  Pref : Inport
  Wref : Inport  Port=2
  " Iabc (pu)" : Scope  Commented=on
  AC1A Excitation System : sps_avr/AC1A Excitation System  Tr=20e-3  KaTa=[400 0.02]  VAminmax=[-14.5 14.5]  VRminmax=[-5.43 6.03]  KfTf=[0.03 1.0]  TbTc=[0 0]  KeTe=[1.0 0.80]  Ve12=[4.18 3.14]  SeVe12=[0.10 0.03]  Kd=0.38  Kc=0.20  v0=[1 1]  TsBlock=0
      settings: SourceProductBaseCode=PS
  Abs : Abs
  Abs1 : Abs
  Add : Sum
  Bus Selector1 : BusSelector  OutputSignals="dq0 components.Field current  ifd (pu)"  OutputAsBus=on
  Bus Selector3 : BusSelector  OutputSignals="dq0 components.Stator voltage  vq (pu),dq0 components.Stator voltage  vd (pu),Mechanical.Rotor speed  wm  (pu),Mechanical.Rotor speed deviation  dw (pu),Output active power   Peo (pu),Stator current"
  Bus Selector7 : BusSelector  OutputSignals="dq0 components.Stator voltage  vd (pu),dq0 components.Stator voltage  vq (pu)"  OutputAsBus=on
  Constant : Constant
  Constant1 : Constant  Value=-1
  Constant2 : Constant  Value=FS_PSH.Turb_enable
  Divide : Product  Inputs=*/
  Fcn3 : Fcn  Expr=sqrt(u(1)^2 + u(2)^2)
  Gain1 : Gain  Gain=FS_PSH.KI
  Gain2 : Gain  Gain=1/FS_PSH.Sn
  Gate Control : Scope  Commented=on
  Gate Governor : Scope  Commented=on
  Gate Position Turb : Scope
  Governor : Subsystem
  Ground2 : Ground
  Ifd : Scope  Commented=on
  Integrator : Integrator
  Output active power (pu) : Scope  Commented=on
  PID Controller1 : pid_lib/PID Controller  Controller=PI  Form=Parallel  TimeDomain=Discrete-time  UseExternalTs=off  SampleTime=Ts  IntegratorMethod=Forward Euler  FilterMethod=Forward Euler  ControllerParametersSource=internal  P=1  I=1/5  D=0  UseFilter=on  N=100  TunerSelectOption=Transfer Function Based (PID Tuner App)  InitialConditionSource=internal  InitialConditionForIntegrator=0  InitialConditionForFilter=0  DifferentiatorICPrevScaledInput=0  ExternalReset=none  TrackingMode=off  Kt=1  LimitOutput=on  SatLimitsSource=internal  UpperSaturationLimit=0.5  LowerSaturationLimit=-0.5  LinearizeAsGain=on  AntiWindupMode=clamping  Kb=1  POutMin=[]  POutMax=[]  IOutMin=[]  IOutMax=[]  DOutMin=[]  DOutMax=[]  NOutMin=[]  NOutMax=[]  SumOutMin=[]  SumOutMax=[]  SaturationOutMin=[]  SaturationOutMax=[]  PParamMin=[]  PParamMax=[]  IParamMin=[]  IParamMax=[]  DParamMin=[]  DParamMax=[]  NParamMin=[]  NParamMax=[]  KbParamMin=[]  KbParamMax=[]  KtParamMin=[]  KtParamMax=[]  KbOutMin=[]  KbOutMax=[]  KtOutMin=[]  KtOutMax=[]  IntegratorOutMin=[]  IntegratorOutMax=[]  FilterOutMin=[]  FilterOutMax=[]  SumI1OutMin=[]  SumI1OutMax=[]  SumI2OutMin=[]  SumI2OutMax=[]  SumI3OutMin=[]  SumI3OutMax=[]  SumI4OutMin=[]  SumI4OutMax=[]  SumDOutMin=[]  SumDOutMax=[]  DifferentiatorOutMin=[]  DifferentiatorOutMax=[]  FilterDiffOutCoefMin=[]  FilterDiffOutCoefMax=[]  ReciprocalOutMin=[]  ReciprocalOutMax=[]  SumDenOutMin=[]  SumDenOutMax=[]  SumNumOutMin=[]  SumNumOutMax=[]  DivideOutMin=[]  DivideOutMax=[]  UdiffTsProdOutMin=[]  UdiffTsProdOutMax=[]  NTsProdOutMin=[]  NTsProdOutMax=[]  UintegralTsProdOutMin=[]  UintegralTsProdOutMax=[]  UngainTsProdOutMin=[]  UngainTsProdOutMax=[]  IntegratorContinuousStateAttributes=''  IntegratorStateMustResolveToSignalObject=off  IntegratorRTWStateStorageClass=Auto  FilterContinuousStateAttributes=''  FilterStateMustResolveToSignalObject=off  FilterRTWStateStorageClass=Auto  ParallelPVariant=InternalParameters  IdealPVariant=Disabled  IVariant=InternalParameters  DVariant=Disabled  IntegratorVariant=Discrete  SatVariant=Enabled  AWVariant=DiscClampingParallel  PCopyVariant=Disabled  TRVariant=Disabled  FdbkBlocksVariant=Forward  IdealPFdbkVariant=Disabled  SatFdbkVariant=Disabled  DerivativeFilterVariant=Disabled  NVariant=Disabled  NCopyVariant=Disabled_SignalSpec  FilterICVariant=Disabled  IntegratorICVariant=InternalICs  ExternalResetVariant=Disabled  TRSumVariant=Passthrough  SumFdbkVariant=Disabled  SumVariant=Sum_PI  TsampFilterVariant=InternalTs  TsampNgainVariant=Passthrough  TsampIntegralVariant=Passthrough  ExternalSaturationOutDataTypeStr=Inherit: Same as second input
  Product : Product
  Rotor speed deviation (pu) : Scope  Commented=on
  Saturation : Saturate  LowerLimit=0.05
  Saturation1 : Saturate  UpperLimit=1  LowerLimit=0
  Saturation2 : Saturate  UpperLimit=100  LowerLimit=-100
  Scope : Scope  Commented=on
  Scope1 : Scope  Commented=on
  Sum1 : Sum  Inputs=++|
  Sum2 : Sum  Inputs=|+-
  Sum3 : Sum  Inputs=|+-
  Switch1 : Switch  Criteria=u2 > Threshold
  Synchronous Machine 7.2 MVA 13.8 kV1 : powerlib/Machines/Synchronous Machine pu Standard  PresetModel=No  MechanicalLoad=Mechanical power Pm  ShowDetailedParameters=on  RotorType=Salient-pole  Units=per unit standard parameters  MeasurementBus=off  NominalParameters="[ FS_PSH.Sn  FS_PSH.Vn   60 ]"  Reactances1=[ 31 32 33 34 35 36 37 ]  Reactances2="[ 0.92, 0.169, 0.135, 0.510, 0.2,  0.13]"  dAxisTimeConstants=Short-circuit  qAxisTimeConstants=Open-circuit  TimeConstants1=[]  TimeConstants2=[]  TimeConstants3=[]  TimeConstants4=[]  TimeConstants5=[ 4.3, 0.032, 0.05 ]  TimeConstants6=[]  TimeConstants7=[]  TimeConstants8=[]  StatorResistance=2.8544e-3  Mechanical=[ 6 0 2]  PolePairs=2  InitialConditions=[0 -94.2826 0.750185 0.750185 0.750185 -24.943 -144.943 95.057 1.29071]  SetSaturation=off  Saturation=[0.6404,0.7127,0.8441,0.9214,0.9956,1.082,1.19,1.316,1.457;0.7,0.7698,0.8872,0.9466,0.9969,1.046,1.1,1.151,1.201]  LoadFlowParameters=[1 150000000 0 0]  TsPowergui=0  TsBlock=-1  IterativeModel=Trapezoidal non iterative  IterativeDiscreteModel=Trapezoidal non iterative  BusType=PV  Pref=150000000  Qref=0  Qmin=-Inf  Qmax=Inf  PLF=0  QLF=0
      settings: AttributesFormatString=\n\n
  Te : Scope  Commented=on
  Tm : Scope  Commented=on
  Tm Turb : Scope  Commented=on
  Transfer Fcn1 : TransferFcn  Numerator=[FS_PSH.G]  Denominator=[FS_PSH.T 1]
  Transfer Fcn2 : TransferFcn  Denominator=[10 1]
  Turbine : Subsystem
  Vd : Scope  Commented=on
  Vq : Scope  Commented=on
  Vref2 : Constant  Value=1.01
  Vt : Scope  Commented=on
  abs_w : Scope  Commented=on
  dP1 : Scope  Commented=on
  w : Scope
  A1 : PMIOPort  Side=Right
  B1 : PMIOPort  Port=2  Side=Right
  C1 : PMIOPort  Port=3  Side=Right
  wires:
  Governor/1(z (Gate Position)) -> [gate_setpoint_governor], Gate Governor/1
  [Wref] -> Governor/1(Wref)
  [w] -> Abs/1
  Add/1 -> Saturation/1
  Saturation/1 -> Turbine/1("z (Gate Position) "), Gate Position Turb/1
  [w] -> Turbine/2(w)
  [Wref] -> Turbine/3(Wref)
  Turbine/1(Tmech) -> Sum1/2, Tm Turb/1
  [dP] -> Sum1/1
  Sum1/1 -> Saturation1/1
  Constant2/1 -> Switch1/2
  Switch1/1 -> Transfer Fcn1/1
  Transfer Fcn1/1 -> Tm/1, Product/2
  Bus Selector3/3 -> [w], w/1  "<Rotor speed  wm  (pu)>"
  Bus Selector3/4 -> [Dw], Rotor speed deviation (pu)/1  "<Rotor speed deviation  dw (pu)>"
  Bus Selector3/5 -> Output active power (pu)/1, [Peo]  "<Output active power   Peo (pu)>"
  Sum2/1 -> Scope/1, PID Controller1/1
  [Pset_pu] -> Sum2/1
  [w] -> Sum3/1
  Constant/1 -> Sum3/2
  Sum3/1 -> Gain1/1
  Gain1/1 -> Integrator/1
  Integrator/1 -> Saturation2/1
  [w] -> Product/1
  Abs/1 -> abs_w/1, Governor/2(w)
  Saturation2/1 -> [dP], dP1/1
  Transfer Fcn2/1 -> [gate_setpoint_control], Gate Control/1
  [gate_setpoint_control] -> Add/1
  [gate_setpoint_governor] -> Add/2
  Product/1 -> [Turb_Power]
  Synchronous Machine 7.2 MVA 13.8 kV1/1 -> [m]
  [Turb_Power] -> Synchronous Machine 7.2 MVA 13.8 kV1/1
  Bus Selector3/2 -> Vd/1, [Vd]  "<Stator voltage  vd (pu)>"
  [m] -> Bus Selector3/1
  Bus Selector3/6 -> " Iabc (pu)"/1, [Iabc]  "<Stator current>"
  Bus Selector3/1 -> Vq/1, [Vq]  "<Stator voltage  vq (pu)>"
  Wref/1 -> [Wref]
  Gain2/1 -> [Pset_pu]
  Pref/1 -> Gain2/1
  Bus Selector7/1 -> Fcn3/1  "Vd Vq"
  Bus Selector1/1 -> Ifd/1, AC1A Excitation System/3  "Ifd"
  [m] -> Bus Selector1/1, Bus Selector7/1
  AC1A Excitation System/1 -> Synchronous Machine 7.2 MVA 13.8 kV1/2
  Fcn3/1 -> Vt/1, AC1A Excitation System/2  "Vt"
  Vref2/1 -> AC1A Excitation System/1
  Ground2/1 -> AC1A Excitation System/4
  [Peo] -> Divide/1
  [w] -> Divide/2
  Divide/1 -> Te/1, [Te]
  PID Controller1/1 -> Scope1/1, Transfer Fcn2/1
  [Te] -> Abs1/1
  Abs1/1 -> Sum2/2
  Constant1/1 -> Switch1/3
  Saturation1/1 -> Switch1/1
  connections:
  Synchronous Machine 7.2 MVA 13.8 kV1/RConn3 -- C1/RConn1
  Synchronous Machine 7.2 MVA 13.8 kV1/RConn2 -- B1/RConn1
  Synchronous Machine 7.2 MVA 13.8 kV1/RConn1 -- A1/RConn1

== system model_FS_PSH_IEEE39/SS_NorthSystem2/GT 10 ==
  5 MW : powerlib/Elements/Three-Phase Parallel RLC Load  LConnTagsString=A|B|C  Configuration=Y (grounded)  NominalVoltage=22e3  Vabc=[1e3 1e3 1e3]  Vabcp=[1e3 1e3 1e3]  NominalFrequency=fNom  UnbalancedPower=off  ActivePower=5e6  InductivePower=0  CapacitivePower=0  Pabc=[10e3 9e3 11e3]  QLabc=[100 90 110]  QCabc=[100 90 110]  Pabcp=[10e3 9e3 11e3]  QLabcp=[100 90 110]  QCabcp=[100 90 110]  Measurements=None  LoadType=constant Z
  Bus Selector1 : BusSelector  OutputSignals="dq0 components.Stator voltage  vq (pu),dq0 components.Stator voltage  vd (pu),Mechanical.Rotor speed  wm  (pu),Mechanical.Rotor speed deviation  dw (pu),Output active power   Peo (pu),Output reactive power  Qeo (pu)"
  Bus 30 : powerlib/Measurements/Three-Phase V-I Measurement  VoltageMeasurement=phase-to-ground  SetLabelV=on  LabelV=V_bus_G10  Vpu=off  VpuLL=off  CurrentMeasurement=no  SetLabelI=on  LabelI=I_bus_G10  Ipu=off  Pbase=100e6  Vbase=16.5e3  OutputType=Complex  PhasorSimulation=off  PSBequivalent=0
  Excitation System : sps_avr/Excitation System  tr=20e-3  reg=[ 200, 0.02 ]  exc=[ 1, 0 .19]  tgr=[ 0, 0 ]  damp=[ 0.0012, 1 ]  sat=[ 0, 0 ]  lim=[ 0, 7.32, 0 ]  v0=[1.025 1.2732]
      settings: SourceProductBaseCode=PS
  GT1_CB14 : Subsystem
  Ground : Ground
  HTG : powerlib/Machines/Hydraulic Turbine and Governor  sm="[ 10/3  0.07 ]"  gate="[  0.01  0.97518  -0.1  0.1 ]"  reg="[  Rp  1.163  0.105  0  0.01  ]"  hyd="[  0  2.67  ]"  dref=0  po=0.324
      settings: SourceProductBaseCode=PS
  Load Flow Bus : powerlib/Measurements/Load Flow Bus  LConnTagsString=a  Phases=single  Connectors=on one side  ID=Bus-30  Vbase=22000  Vref=1.025  Vangle=0  VLF=1.025  VLFb=1  VLFc=1  angleLF=-2.488  angleLFb=0  angleLFc=0
      settings: AttributesFormatString=%<ID>\n%<Vbase>V\n%<VLF>pu\n%<angleLF>deg.
  Machine 10 1000 MVA 22 kV : powerlib/Machines/Synchronous Machine pu Standard  PresetModel=No  MechanicalLoad=Mechanical power Pm  ShowDetailedParameters=on  RotorType=Round  Units=per unit standard parameters  MeasurementBus=off  NominalParameters="[ 1000E6  22000   fNom]"  Reactances1="[ 1.29 0.4 0.2 0.89 0.103 0.2 0.013  ]"  Reactances2=[ 0.995, 0.195, 0.155, 0.568, 0.143, 0.16 ]  dAxisTimeConstants=Open-circuit  qAxisTimeConstants=Open-circuit  TimeConstants1=[]  TimeConstants2=[10.2 0.03 0.02 0.04]  TimeConstants3=[]  TimeConstants4=[]  TimeConstants5=[ 9.2, 0.01, 0.01 ]  TimeConstants6=[]  TimeConstants7=[]  TimeConstants8=[]  StatorResistance=0.005  Mechanical=[ 3.255 0.02 20]  PolePairs=20  InitialConditions=[0 -77.6756 0.367118 0.367118 0.367118 -24.0341 -144.034 95.9659 1.27317]  SetSaturation=off  Saturation=[0.6404,0.7127,0.8441,0.9214,0.9956,1.082,1.19,1.316,1.457;0.7,0.7698,0.8872,0.9466,0.9969,1.046,1.1,1.151,1.201]  LoadFlowParameters=[1 632000000 21938.4 0]  TsPowergui=0  TsBlock=-1  IterativeModel=Trapezoidal non iterative  IterativeDiscreteModel=Trapezoidal non iterative  BusType=PV  Pref=3.5e+008  Qref=0  Qmin=-500e6  Qmax=200e6  PLF=0  QLF=0
      settings: AttributesFormatString=\n\n
  Pref : Constant  Value=0.324
  Terminator5 : Terminator
  Transformer 10 1419 MVA 22 kV / 345 kV : powerlib/Elements/Three-Phase Transformer (Two Windings)  Winding1Connection=Delta (D1)  Winding2Connection=Yg  CoreType=Three single-phase transformers  SetSaturation=off  Hysteresis=off  DataFile='hysteresis'  SetInitialFlux=off  Measurements=None  UNITS=pu  NominalPower=[ 1419e6 fNom]  Winding1="[ 22e3   0    0.0181*1419/100/2 ]"  Winding2=|  Rm=500  Lm=500  L0=0.5  Saturation="[ 0,0  ;  0.005,1.2  ;  1.0,1.4 ]"  InitialFluxes=[ 0.8 , -0.8 , 0.7 ]  BreakLoop=off  DiscreteSolver=Trapezoidal iterative  DataType=off  TransfoNumber=0
      | [ 1.025*345e3 0    0.0181*1419/100/2
      | ]
  Vref : Constant  Value=1.025
  wref : Constant
  A : PMIOPort  Side=Right
  B : PMIOPort  Port=2  Side=Right
  C : PMIOPort  Port=3  Side=Right
  tag scope: P_G10=global, Q_G10=global, V_G10=global, Wm_G10=global
  wires:
  Ground/1 -> Excitation System/4
  HTG/2 -> Terminator5/1
  Vref/1 -> Excitation System/1
  Pref/1 -> HTG/2
  wref/1 -> HTG/1
  Excitation System/1 -> Machine 10 1000 MVA 22 kV/2
  HTG/1 -> Machine 10 1000 MVA 22 kV/1
  Machine 10 1000 MVA 22 kV/1 -> Bus Selector1/1
  Bus Selector1/1 -> Excitation System/3  "<Stator voltage  vq (pu)>"
  Bus Selector1/2 -> Excitation System/2  "<Stator voltage  vd (pu)>"
  Bus Selector1/3 -> HTG/3, [Wm_G10]  "<Rotor speed  wm  (pu)>"
  Bus Selector1/4 -> HTG/5  "<Rotor speed deviation  dw (pu)>"
  Bus Selector1/5 -> HTG/4, [P_G10]  "<Output active power   Peo (pu)>"
  Bus Selector1/6 -> [Q_G10]  "<Output reactive power  Qeo (pu)>"
  [V_bus_G10] -> [V_G10]
  connections:
  Transformer 10 1419 MVA 22 kV / 345 kV/LConn1 -- Load Flow Bus/LConn1 -- Bus 30/RConn1 -- 5 MW/LConn1
  Transformer 10 1419 MVA 22 kV / 345 kV/LConn2 -- Bus 30/RConn2 -- 5 MW/LConn2
  Transformer 10 1419 MVA 22 kV / 345 kV/LConn3 -- Bus 30/RConn3 -- 5 MW/LConn3
  Machine 10 1000 MVA 22 kV/RConn1 -- Bus 30/LConn1
  Machine 10 1000 MVA 22 kV/RConn2 -- Bus 30/LConn2
  Machine 10 1000 MVA 22 kV/RConn3 -- Bus 30/LConn3
  GT1_CB14/LConn1 -- Transformer 10 1419 MVA 22 kV / 345 kV/RConn1
  GT1_CB14/LConn2 -- Transformer 10 1419 MVA 22 kV / 345 kV/RConn2
  GT1_CB14/LConn3 -- Transformer 10 1419 MVA 22 kV / 345 kV/RConn3
  A/RConn1 -- GT1_CB14/RConn1
  C/RConn1 -- GT1_CB14/RConn3
  B/RConn1 -- GT1_CB14/RConn2

== system model_FS_PSH_IEEE39/SS_NorthSystem2/Load 18 ==
  Bus_L18 : powerlib/Measurements/Three-Phase V-I Measurement  VoltageMeasurement=phase-to-ground  SetLabelV=off  LabelV=V_Bus_L18  Vpu=off  VpuLL=off  CurrentMeasurement=yes  SetLabelI=on  LabelI=I_L18  Ipu=off  Pbase=100e6  Vbase=230e3  OutputType=Complex  PhasorSimulation=off  PSBequivalent=0
  Terminator : Terminator
  Three-Phase Dynamic Load : powerlib/Elements/Three-Phase Dynamic Load  NominalVoltage=[345e3 fNom]  ActiveReactivePowers=[1.58e+08 3e+07]  PositiveSequence=[1.0086 19.7218]  ExternalControl=on  NpNq=[0 0]  TimeConstants="[0  0  0  0]"  MinimumVoltage=0.7  Tfilter=1e-4  LoadFlowParameters=[4,0,0,0,0]
      settings: SourceProductBaseCode=PS
  A : PMIOPort  Side=Left
  B : PMIOPort  Port=2  Side=Left
  C : PMIOPort  Port=3  Side=Left
  tag scope: V_L18=global
  wires:
  Three-Phase Dynamic Load/1 -> Terminator/1
  Bus_L18/1 -> [V_L18]
  [load18] -> Three-Phase Dynamic Load/1
  connections:
  Bus_L18/RConn3 -- Three-Phase Dynamic Load/LConn3
  Bus_L18/RConn2 -- Three-Phase Dynamic Load/LConn2
  A/RConn1 -- Bus_L18/LConn1
  B/RConn1 -- Bus_L18/LConn2
  C/RConn1 -- Bus_L18/LConn3
  Bus_L18/RConn1 -- Three-Phase Dynamic Load/LConn1
